simulink model "dieukhien"  (R2019a)
settings: Solver=VariableStepAuto  StartTime=0.0  StopTime=10  RelTol=1e-3
settings Model: Creator=dell  LastModifiedBy=dell

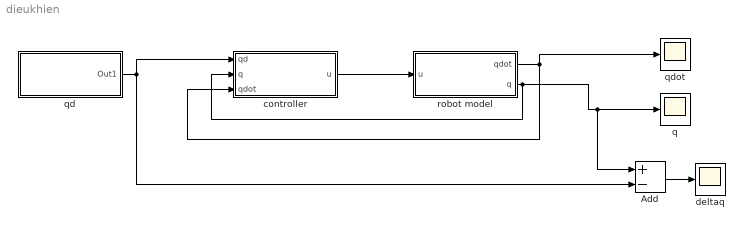
== system dieukhien ==
  Add : Sum  Inputs=+-
  controller : Subsystem
  deltaq : Scope
  "q " : Scope
  qd : Subsystem
  qdot : Scope
  robot model : Subsystem
  wires:
  qd/1(Out1) -> controller/1(qd), Add/2
  controller/1("u ") -> robot model/1(u)
  robot model/1(qdot) -> controller/3(qdot), qdot/1
  robot model/2("q ") -> controller/2(q), Add/1, "q "/1
  Add/1 -> deltaq/1

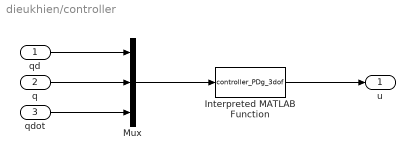
== system dieukhien/controller ==
  qd : Inport
  q : Inport  Port=2
  qdot : Inport  Port=3
  Interpreted MATLAB Function : MATLABFcn  MATLABFcn=controller_PDg_3dof
  Mux : Mux  Inputs=3
  "u " : Outport
  wires:
  Mux/1 -> Interpreted MATLAB Function/1
  qd/1 -> Mux/1
  Interpreted MATLAB Function/1 -> "u "/1
  q/1 -> Mux/2
  qdot/1 -> Mux/3

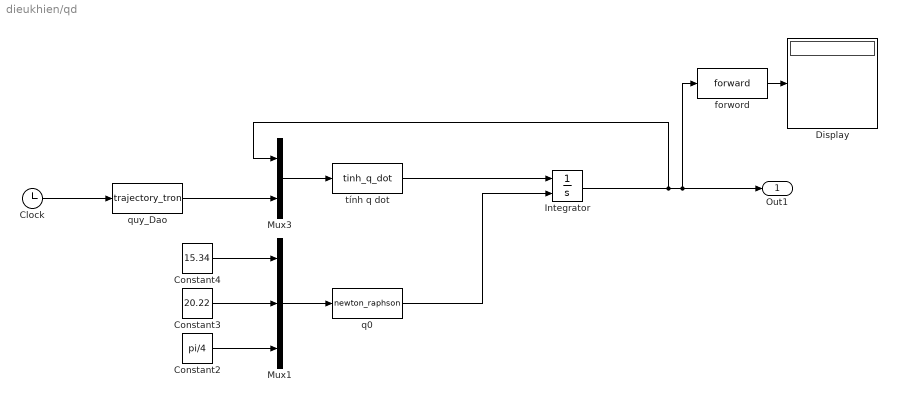
== system dieukhien/qd ==
  Clock : Clock
  Constant2 : Constant  Value=pi/4
  Constant3 : Constant  Value=20.22
  Constant4 : Constant  Value=15.34
  Display : Display
      settings: Decimation=3
  Integrator : Integrator  InitialConditionSource=external
  Mux1 : Mux  Inputs=3
  Mux3 : Mux  Inputs=2
  forword : MATLABFcn  MATLABFcn=forward  OutputDimensions=3
  q0 : MATLABFcn  MATLABFcn=newton_raphson  OutputDimensions=3
  quy_Dao : MATLABFcn  MATLABFcn=trajectory_tron  OutputDimensions=6
  "tính q dot " : MATLABFcn  MATLABFcn=tinh_q_dot  OutputDimensions=3
  Out1 : Outport
  wires:
  Constant3/1 -> Mux1/2
  Constant2/1 -> Mux1/3
  q0/1 -> Integrator/2
  Clock/1 -> quy_Dao/1
  "tính q dot "/1 -> Integrator/1
  Constant4/1 -> Mux1/1
  Mux1/1 -> q0/1
  Integrator/1 -> Mux3/1, forword/1, Out1/1
  quy_Dao/1 -> Mux3/2
  Mux3/1 -> "tính q dot "/1
  forword/1 -> Display/1

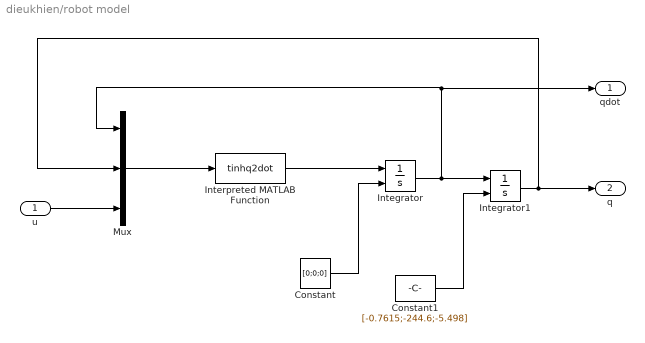
== system dieukhien/robot model ==
  u : Inport
  Constant : Constant  Value=[0;0;0]
  Constant1 : Constant  Value=[-0.7615;-244.6;-5.498]
  Integrator : Integrator  InitialConditionSource=external
  Integrator1 : Integrator  InitialConditionSource=external
  Interpreted MATLAB Function : MATLABFcn  MATLABFcn=tinhq2dot
  Mux : Mux  Inputs=3
  qdot : Outport
  "q " : Outport  Port=2
  wires:
  Mux/1 -> Interpreted MATLAB Function/1
  Integrator/1 -> Mux/1, qdot/1, Integrator1/1
  u/1 -> Mux/3
  Integrator1/1 -> Mux/2, "q "/1
  Interpreted MATLAB Function/1 -> Integrator/1
  Constant/1 -> Integrator/2
  Constant1/1 -> Integrator1/2
